simulink model "ctrl_custom"  (R2016b)
settings: Solver=ode3  StartTime=0.0  StopTime=inf  FixedStep=0.01  RelTol=1e-3  EnableMultiTasking=on
undefined symbols (not defined in the file): C, D, DiscIntNeverNeededParam, eps_c, epsilon, hd, hd2, I_s, k_cc, K_omega, K_q1f, K_q1r, K_q2f, K_q2r, K_q3f, K_q3r, K_q4f, K_q4r, K_q5f, K_q5r, K_q6f, K_q6r, K_T1f, K_T1r, K_T2f, K_T2r, K_T3f, K_T3r, K_T4f, K_T4r, K_T5f, K_T5r, K_T6f, K_T6r, Kp, Max_Acceleration, Max_rotation, Max_thrust, Min_thrust, n_c, n_max, p_cc, pwm_thr1_backward, pwm_thr1_forward, pwm_thr2_backward, pwm_thr2_forward, pwm_thr3_backward, pwm_thr3_forward, pwm_thr4_backward, pwm_thr4_forward, pwm_thr5_backward, pwm_thr5_forward, pwm_thr6_backward, pwm_thr6_forward, Q_f0, Q_max, r_cc, Rho, Thruster
libraries: dspmtrx3 x10, marine_gnc x8, simulink x7, simulink_extras x3
(part 4 of 6)

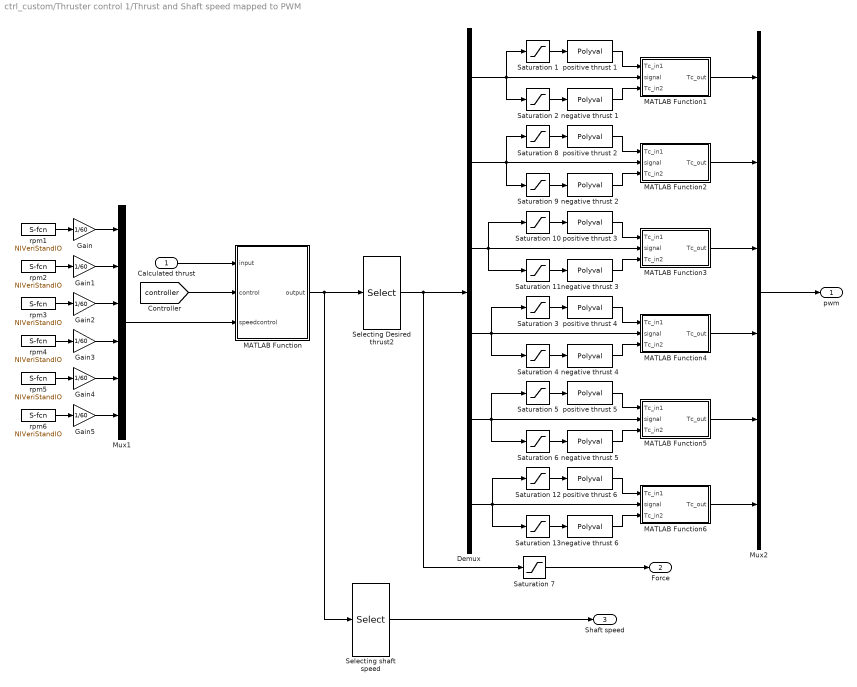
== system ctrl_custom/Thruster control 1/Thrust and Shaft speed mapped to PWM ==
  Calculated thrust : Inport
  Demux : Demux  Outputs=6
  Gain{,1..5} (6 alike) : Gain  Gain=1/60
  MATLAB Function : MATLAB Function  TreatAsAtomicUnit=on
  MATLAB Function1 : MATLAB Function  TreatAsAtomicUnit=on
  MATLAB Function2 : MATLAB Function  TreatAsAtomicUnit=on
  MATLAB Function3 : MATLAB Function  TreatAsAtomicUnit=on
  MATLAB Function4 : MATLAB Function  TreatAsAtomicUnit=on
  MATLAB Function5 : MATLAB Function  TreatAsAtomicUnit=on
  MATLAB Function6 : MATLAB Function  TreatAsAtomicUnit=on
  Mux1 : Mux  Inputs=6
  Mux2 : Mux  Inputs=6
  Saturation {1,3,5,8,10,12} (6 alike) : Saturate  UpperLimit=Max_thrust  LowerLimit=0
  Saturation {2,4,6,9,11,13} (6 alike) : Saturate  UpperLimit=0  LowerLimit=Min_thrust
  Saturation 7 : Saturate  UpperLimit=Max_thrust  LowerLimit=-Max_thrust
  Selecting Desired thrust2 : Selector  InputPortWidth=12  IndexOptions=Index vector (dialog)  Indices=[1 3 5 7 9 11]  OutputSizes=1
  Selecting shaft speed : Selector  InputPortWidth=12  IndexOptions=Index vector (dialog)  Indices=[2 4 6 8 10 12]  OutputSizes=1
  negative thrust 1 : Polyval  Coefs=pwm_thr1_backward
  negative thrust 2 : Polyval  Coefs=pwm_thr2_backward
  negative thrust 3 : Polyval  Coefs=pwm_thr3_backward
  negative thrust 4 : Polyval  Coefs=pwm_thr4_backward
  negative thrust 5 : Polyval  Coefs=pwm_thr5_backward
  negative thrust 6 : Polyval  Coefs=pwm_thr6_backward
  positive thrust 1 : Polyval  Coefs=pwm_thr1_forward
  positive thrust 2 : Polyval  Coefs=pwm_thr2_forward
  positive thrust 3 : Polyval  Coefs=pwm_thr3_forward
  positive thrust 4 : Polyval  Coefs=pwm_thr4_forward
  positive thrust 5 : Polyval  Coefs=pwm_thr5_forward
  positive thrust 6 : Polyval  Coefs=pwm_thr6_forward
  "rpm1 " : S-Function  Priority=1  FunctionName=NIVeriStandIO  Parameters=width dtype portnum stime stype btype  SFunctionDeploymentMode=off  EnableBusSupport=off  mask(NI VeriStand Inport){portnum=1, width=-1, stime=-1, dtype=auto, stype=auto, btype=1}
      mask prompts: portnum "Port number:"; width "Port dimensions (-1 for dynamically sized):"; stime "Sample time (-1 for inherited):"; dtype "Data type:"; stype "Signal type:"; btype "Block type:"
      mask help: Use this inport on any level of nested subsystems to allow NI VeriStand software to map signals to it.
      mask init:
      | NIVeriStandIO_init;
      settings: CopyFcn=NIVeriStand_MDL_functions('', 'IO_copy');  DeleteFcn=NIVeriStand_MDL_functions('', 'IO_delete');  MoveFcn=set_param(gcb, 'Mask', 'on');
      mask Callback portnum: NIVeriStand_MDL_functions('', 'IO_setportnum');
      mask TypeOptions dtype: auto | double | single | int8 | uint8 | int16 | uint16 | int32 | uint32 | boolean
      mask Callback dtype: NIVeriStand_MDL_functions('', 'IO_booleansignal');
      mask TypeOptions stype: auto | real | complex
      mask Display:
      | patch([-x x], [-y y], [.90980 .81960 .32156]);
      | plot([xrad -x x xrad], [yrad -y y yrad]);
      | fprintf('NI In%d', portnum);
  rpm2 : S-Function  Priority=2  FunctionName=NIVeriStandIO  Parameters=width dtype portnum stime stype btype  SFunctionDeploymentMode=off  EnableBusSupport=off  mask(NI VeriStand Inport){portnum=2, width=-1, stime=-1, dtype=auto, stype=auto, btype=1}
      mask prompts: portnum "Port number:"; width "Port dimensions (-1 for dynamically sized):"; stime "Sample time (-1 for inherited):"; dtype "Data type:"; stype "Signal type:"; btype "Block type:"
      mask help: Use this inport on any level of nested subsystems to allow NI VeriStand software to map signals to it.
      mask init:
      | NIVeriStandIO_init;
      settings: CopyFcn=NIVeriStand_MDL_functions('', 'IO_copy');  DeleteFcn=NIVeriStand_MDL_functions('', 'IO_delete');  MoveFcn=set_param(gcb, 'Mask', 'on');
      mask Callback portnum: NIVeriStand_MDL_functions('', 'IO_setportnum');
      mask TypeOptions dtype: auto | double | single | int8 | uint8 | int16 | uint16 | int32 | uint32 | boolean
      mask Callback dtype: NIVeriStand_MDL_functions('', 'IO_booleansignal');
      mask TypeOptions stype: auto | real | complex
      mask Display:
      | patch([-x x], [-y y], [.90980 .81960 .32156]);
      | plot([xrad -x x xrad], [yrad -y y yrad]);
      | fprintf('NI In%d', portnum);
  rpm3 : S-Function  Priority=3  FunctionName=NIVeriStandIO  Parameters=width dtype portnum stime stype btype  SFunctionDeploymentMode=off  EnableBusSupport=off  mask(NI VeriStand Inport){portnum=3, width=-1, stime=-1, dtype=auto, stype=auto, btype=1}
      mask prompts: portnum "Port number:"; width "Port dimensions (-1 for dynamically sized):"; stime "Sample time (-1 for inherited):"; dtype "Data type:"; stype "Signal type:"; btype "Block type:"
      mask help: Use this inport on any level of nested subsystems to allow NI VeriStand software to map signals to it.
      mask init:
      | NIVeriStandIO_init;
      settings: CopyFcn=NIVeriStand_MDL_functions('', 'IO_copy');  DeleteFcn=NIVeriStand_MDL_functions('', 'IO_delete');  MoveFcn=set_param(gcb, 'Mask', 'on');
      mask Callback portnum: NIVeriStand_MDL_functions('', 'IO_setportnum');
      mask TypeOptions dtype: auto | double | single | int8 | uint8 | int16 | uint16 | int32 | uint32 | boolean
      mask Callback dtype: NIVeriStand_MDL_functions('', 'IO_booleansignal');
      mask TypeOptions stype: auto | real | complex
      mask Display:
      | patch([-x x], [-y y], [.90980 .81960 .32156]);
      | plot([xrad -x x xrad], [yrad -y y yrad]);
      | fprintf('NI In%d', portnum);
  rpm4 : S-Function  Priority=4  FunctionName=NIVeriStandIO  Parameters=width dtype portnum stime stype btype  SFunctionDeploymentMode=off  EnableBusSupport=off  mask(NI VeriStand Inport){portnum=4, width=-1, stime=-1, dtype=auto, stype=auto, btype=1}
      mask prompts: portnum "Port number:"; width "Port dimensions (-1 for dynamically sized):"; stime "Sample time (-1 for inherited):"; dtype "Data type:"; stype "Signal type:"; btype "Block type:"
      mask help: Use this inport on any level of nested subsystems to allow NI VeriStand software to map signals to it.
      mask init:
      | NIVeriStandIO_init;
      settings: CopyFcn=NIVeriStand_MDL_functions('', 'IO_copy');  DeleteFcn=NIVeriStand_MDL_functions('', 'IO_delete');  MoveFcn=set_param(gcb, 'Mask', 'on');
      mask Callback portnum: NIVeriStand_MDL_functions('', 'IO_setportnum');
      mask TypeOptions dtype: auto | double | single | int8 | uint8 | int16 | uint16 | int32 | uint32 | boolean
      mask Callback dtype: NIVeriStand_MDL_functions('', 'IO_booleansignal');
      mask TypeOptions stype: auto | real | complex
      mask Display:
      | patch([-x x], [-y y], [.90980 .81960 .32156]);
      | plot([xrad -x x xrad], [yrad -y y yrad]);
      | fprintf('NI In%d', portnum);
  rpm5 : S-Function  Priority=5  FunctionName=NIVeriStandIO  Parameters=width dtype portnum stime stype btype  SFunctionDeploymentMode=off  EnableBusSupport=off  mask(NI VeriStand Inport){portnum=5, width=-1, stime=-1, dtype=auto, stype=auto, btype=1}
      mask prompts: portnum "Port number:"; width "Port dimensions (-1 for dynamically sized):"; stime "Sample time (-1 for inherited):"; dtype "Data type:"; stype "Signal type:"; btype "Block type:"
      mask help: Use this inport on any level of nested subsystems to allow NI VeriStand software to map signals to it.
      mask init:
      | NIVeriStandIO_init;
      settings: CopyFcn=NIVeriStand_MDL_functions('', 'IO_copy');  DeleteFcn=NIVeriStand_MDL_functions('', 'IO_delete');  MoveFcn=set_param(gcb, 'Mask', 'on');
      mask Callback portnum: NIVeriStand_MDL_functions('', 'IO_setportnum');
      mask TypeOptions dtype: auto | double | single | int8 | uint8 | int16 | uint16 | int32 | uint32 | boolean
      mask Callback dtype: NIVeriStand_MDL_functions('', 'IO_booleansignal');
      mask TypeOptions stype: auto | real | complex
      mask Display:
      | patch([-x x], [-y y], [.90980 .81960 .32156]);
      | plot([xrad -x x xrad], [yrad -y y yrad]);
      | fprintf('NI In%d', portnum);
  rpm6 : S-Function  Priority=6  FunctionName=NIVeriStandIO  Parameters=width dtype portnum stime stype btype  SFunctionDeploymentMode=off  EnableBusSupport=off  mask(NI VeriStand Inport){portnum=6, width=-1, stime=-1, dtype=auto, stype=auto, btype=1}
      mask prompts: portnum "Port number:"; width "Port dimensions (-1 for dynamically sized):"; stime "Sample time (-1 for inherited):"; dtype "Data type:"; stype "Signal type:"; btype "Block type:"
      mask help: Use this inport on any level of nested subsystems to allow NI VeriStand software to map signals to it.
      mask init:
      | NIVeriStandIO_init;
      settings: CopyFcn=NIVeriStand_MDL_functions('', 'IO_copy');  DeleteFcn=NIVeriStand_MDL_functions('', 'IO_delete');  MoveFcn=set_param(gcb, 'Mask', 'on');
      mask Callback portnum: NIVeriStand_MDL_functions('', 'IO_setportnum');
      mask TypeOptions dtype: auto | double | single | int8 | uint8 | int16 | uint16 | int32 | uint32 | boolean
      mask Callback dtype: NIVeriStand_MDL_functions('', 'IO_booleansignal');
      mask TypeOptions stype: auto | real | complex
      mask Display:
      | patch([-x x], [-y y], [.90980 .81960 .32156]);
      | plot([xrad -x x xrad], [yrad -y y yrad]);
      | fprintf('NI In%d', portnum);
  pwm : Outport
  Force : Outport  Port=2
  "Shaft speed " : Outport  Port=3
  wires:
  MATLAB Function/1(output) -> Selecting shaft speed/1, Selecting Desired thrust2/1
  [controller] -> MATLAB Function/2(control)
  Mux2/1 -> pwm/1
  Selecting Desired thrust2/1 -> Saturation 7/1, Demux/1
  Selecting shaft speed/1 -> "Shaft speed "/1
  Saturation 7/1 -> Force/1
  "rpm1 "/1 -> Gain/1
  rpm2/1 -> Gain1/1
  rpm3/1 -> Gain2/1
  rpm4/1 -> Gain3/1
  rpm5/1 -> Gain4/1
  rpm6/1 -> Gain5/1
  Mux1/1 -> MATLAB Function/3(speedcontrol)
  positive thrust 1/1 -> MATLAB Function1/1(Tc_in1)
  negative thrust 1/1 -> MATLAB Function1/3(Tc_in2)
  Demux/1 -> Saturation 1/1, MATLAB Function1/2(signal), Saturation 2/1
  MATLAB Function1/1(Tc_out) -> Mux2/1
  Saturation 1/1 -> positive thrust 1/1
  Saturation 2/1 -> negative thrust 1/1
  positive thrust 2/1 -> MATLAB Function2/1(Tc_in1)
  negative thrust 2/1 -> MATLAB Function2/3(Tc_in2)
  Demux/2 -> Saturation 9/1, Saturation 8/1, MATLAB Function2/2(signal)
  MATLAB Function2/1(Tc_out) -> Mux2/2
  Saturation 8/1 -> positive thrust 2/1
  Saturation 9/1 -> negative thrust 2/1
  positive thrust 3/1 -> MATLAB Function3/1(Tc_in1)
  negative thrust 3/1 -> MATLAB Function3/3(Tc_in2)
  Demux/3 -> Saturation 11/1, MATLAB Function3/2(signal), Saturation 10/1
  MATLAB Function3/1(Tc_out) -> Mux2/3
  Saturation 10/1 -> positive thrust 3/1
  Saturation 11/1 -> negative thrust 3/1
  positive thrust 4/1 -> MATLAB Function4/1(Tc_in1)
  negative thrust 4/1 -> MATLAB Function4/3(Tc_in2)
  MATLAB Function4/1(Tc_out) -> Mux2/4
  Saturation 3/1 -> positive thrust 4/1
  Saturation 4/1 -> negative thrust 4/1
  Demux/4 -> Saturation 3/1, Saturation 4/1, MATLAB Function4/2(signal)
  positive thrust 5/1 -> MATLAB Function5/1(Tc_in1)
  negative thrust 5/1 -> MATLAB Function5/3(Tc_in2)
  MATLAB Function5/1(Tc_out) -> Mux2/5
  Saturation 5/1 -> positive thrust 5/1
  Saturation 6/1 -> negative thrust 5/1
  Demux/5 -> Saturation 5/1, MATLAB Function5/2(signal), Saturation 6/1
  positive thrust 6/1 -> MATLAB Function6/1(Tc_in1)
  negative thrust 6/1 -> MATLAB Function6/3(Tc_in2)
  MATLAB Function6/1(Tc_out) -> Mux2/6
  Saturation 12/1 -> positive thrust 6/1
  Saturation 13/1 -> negative thrust 6/1
  Demux/6 -> Saturation 13/1, Saturation 12/1, MATLAB Function6/2(signal)
  Gain/1 -> Mux1/1
  Gain5/1 -> Mux1/6
  Gain4/1 -> Mux1/5
  Gain3/1 -> Mux1/4
  Gain2/1 -> Mux1/3
  Gain1/1 -> Mux1/2
  Calculated thrust/1 -> MATLAB Function/1(input)

== system ctrl_custom/Thruster control 1/Thruster 1 ==
  Desired thrust 1 : Inport
  shaft speed : Inport  Port=2
  Constant : Constant  Value=hd2.den{1,1}
  Constant1 : Constant  Value=hd2.num{1,1}
  Delay : Delay  DelayLength=1  InitialCondition=0
  Discrete Transfer Fcn : DiscreteTransferFcn  NumeratorSource=Input port  DenominatorSource=Input port  Denominator=[0.2 1]  SampleTime=0.01  a0EqualsOne=on
      settings: InputPortMap=u0,p1,p3
  Losses (placeholder) : Constant  Value=0
  Propeller Hydrodynamics : Subsystem
  Shaft dynamics : Subsystem
  Thruster control : Subsystem
  "Commanded thrust " : Outport
  Shaft speed : Outport  Port=2
  wires:
  Losses (placeholder)/1 -> Propeller Hydrodynamics/1(env)
  Shaft dynamics/1(n) -> Shaft speed/1, Propeller Hydrodynamics/2(n)
  Propeller Hydrodynamics/2(Qa) -> Delay/1
  Propeller Hydrodynamics/1(Ta) -> "Commanded thrust "/1
  Thruster control/1(Qc) -> Discrete Transfer Fcn/1
  Constant1/1 -> Discrete Transfer Fcn/2
  Constant/1 -> Discrete Transfer Fcn/3
  Discrete Transfer Fcn/1 -> Shaft dynamics/1(Qm)
  shaft speed/1 -> Thruster control/2(n)
  Delay/1 -> Shaft dynamics/2(Qa)
  Desired thrust 1/1 -> Thruster control/1("T_d ")

== system ctrl_custom/Thruster control 1/Thruster 2 ==
  Desired thrust 1 : Inport
  shaft speed : Inport  Port=2
  Constant : Constant  Value=hd2.den{1,1}
  Constant1 : Constant  Value=hd2.num{1,1}
  Delay : Delay  DelayLength=1  InitialCondition=0
  Discrete Transfer Fcn : DiscreteTransferFcn  NumeratorSource=Input port  DenominatorSource=Input port  Denominator=[0.2 1]  SampleTime=0.01  a0EqualsOne=on
      settings: InputPortMap=u0,p1,p3
  Losses (placeholder) : Constant  Value=0
  Propeller Hydrodynamics : Subsystem
  Shaft dynamics : Subsystem
  Thruster control : Subsystem
  "Commanded thrust " : Outport
  Shaft speed : Outport  Port=2
  wires:
  Losses (placeholder)/1 -> Propeller Hydrodynamics/1(env)
  Shaft dynamics/1(n) -> Propeller Hydrodynamics/2(n), Shaft speed/1
  Propeller Hydrodynamics/2(Qa) -> Delay/1
  Thruster control/1(Qc) -> Discrete Transfer Fcn/1
  Discrete Transfer Fcn/1 -> Shaft dynamics/1(Qm)
  Desired thrust 1/1 -> Thruster control/1("T_d ")
  Propeller Hydrodynamics/1(Ta) -> "Commanded thrust "/1
  Constant1/1 -> Discrete Transfer Fcn/2
  Constant/1 -> Discrete Transfer Fcn/3
  shaft speed/1 -> Thruster control/2(n)
  Delay/1 -> Shaft dynamics/2(Qa)

== system ctrl_custom/Thruster control 1/Thruster 3 ==
  Desired thrust 1 : Inport
  shaft speed : Inport  Port=2
  Constant : Constant  Value=hd2.den{1,1}
  Constant1 : Constant  Value=hd2.num{1,1}
  Delay : Delay  DelayLength=1  InitialCondition=0
  Discrete Transfer Fcn : DiscreteTransferFcn  NumeratorSource=Input port  DenominatorSource=Input port  Denominator=[0.2 1]  SampleTime=0.01  a0EqualsOne=on
      settings: InputPortMap=u0,p1,p3
  Losses (placeholder) : Constant  Value=0
  Propeller Hydrodynamics : Subsystem
  Shaft dynamics : Subsystem
  Thruster control : Subsystem
  "Commanded thrust " : Outport
  Shaft speed : Outport  Port=2
  wires:
  Losses (placeholder)/1 -> Propeller Hydrodynamics/1(env)
  Shaft dynamics/1(n) -> Propeller Hydrodynamics/2(n), Shaft speed/1
  Propeller Hydrodynamics/2(Qa) -> Delay/1
  Thruster control/1(Qc) -> Discrete Transfer Fcn/1
  Discrete Transfer Fcn/1 -> Shaft dynamics/1(Qm)
  Desired thrust 1/1 -> Thruster control/1("T_d ")
  Propeller Hydrodynamics/1(Ta) -> "Commanded thrust "/1
  Constant1/1 -> Discrete Transfer Fcn/2
  Constant/1 -> Discrete Transfer Fcn/3
  shaft speed/1 -> Thruster control/2(n)
  Delay/1 -> Shaft dynamics/2(Qa)

== system ctrl_custom/Thruster control 1/Thruster 4 ==
  Desired thrust 1 : Inport
  shaft speed : Inport  Port=2
  Constant : Constant  Value=hd2.den{1,1}
  Constant1 : Constant  Value=hd2.num{1,1}
  Delay : Delay  DelayLength=1  InitialCondition=0
  Discrete Transfer Fcn : DiscreteTransferFcn  NumeratorSource=Input port  DenominatorSource=Input port  Denominator=[0.2 1]  SampleTime=0.01  a0EqualsOne=on
      settings: InputPortMap=u0,p1,p3
  Losses (placeholder) : Constant  Value=0
  Propeller Hydrodynamics : Subsystem
  Shaft dynamics : Subsystem
  Thruster control : Subsystem
  "Commanded thrust " : Outport
  Shaft speed : Outport  Port=2
  wires:
  Losses (placeholder)/1 -> Propeller Hydrodynamics/1(env)
  Shaft dynamics/1(n) -> Propeller Hydrodynamics/2(n), Shaft speed/1
  Propeller Hydrodynamics/2(Qa) -> Delay/1
  Thruster control/1(Qc) -> Discrete Transfer Fcn/1
  Discrete Transfer Fcn/1 -> Shaft dynamics/1(Qm)
  Desired thrust 1/1 -> Thruster control/1("T_d ")
  Propeller Hydrodynamics/1(Ta) -> "Commanded thrust "/1
  Constant1/1 -> Discrete Transfer Fcn/2
  Constant/1 -> Discrete Transfer Fcn/3
  shaft speed/1 -> Thruster control/2(n)
  Delay/1 -> Shaft dynamics/2(Qa)

== system ctrl_custom/Thruster control 1/Thruster 5 ==
  Desired thrust 1 : Inport
  shaft speed : Inport  Port=2
  Constant : Constant  Value=hd2.den{1,1}
  Constant1 : Constant  Value=hd2.num{1,1}
  Delay : Delay  DelayLength=1  InitialCondition=0
  Discrete Transfer Fcn : DiscreteTransferFcn  NumeratorSource=Input port  DenominatorSource=Input port  Denominator=[0.2 1]  SampleTime=0.01  a0EqualsOne=on
      settings: InputPortMap=u0,p1,p3
  Losses (placeholder) : Constant  Value=0
  Propeller Hydrodynamics : Subsystem
  Shaft dynamics : Subsystem
  Thruster control : Subsystem
  "Commanded thrust " : Outport
  Shaft speed : Outport  Port=2
  wires:
  Losses (placeholder)/1 -> Propeller Hydrodynamics/1(env)
  Shaft dynamics/1(n) -> Propeller Hydrodynamics/2(n), Shaft speed/1
  Propeller Hydrodynamics/2(Qa) -> Delay/1
  Thruster control/1(Qc) -> Discrete Transfer Fcn/1
  Discrete Transfer Fcn/1 -> Shaft dynamics/1(Qm)
  Desired thrust 1/1 -> Thruster control/1("T_d ")
  Propeller Hydrodynamics/1(Ta) -> "Commanded thrust "/1
  Constant1/1 -> Discrete Transfer Fcn/2
  Constant/1 -> Discrete Transfer Fcn/3
  shaft speed/1 -> Thruster control/2(n)
  Delay/1 -> Shaft dynamics/2(Qa)

== system ctrl_custom/Thruster control 1/Thruster 6 ==
  Desired thrust 1 : Inport
  shaft speed : Inport  Port=2
  Constant : Constant  Value=hd2.den{1,1}
  Constant1 : Constant  Value=hd2.num{1,1}
  Delay : Delay  DelayLength=1  InitialCondition=0
  Discrete Transfer Fcn : DiscreteTransferFcn  NumeratorSource=Input port  DenominatorSource=Input port  Denominator=[0.2 1]  SampleTime=0.01  a0EqualsOne=on
      settings: InputPortMap=u0,p1,p3
  Losses (placeholder) : Constant  Value=0
  Propeller Hydrodynamics : Subsystem
  Shaft dynamics : Subsystem
  Thruster control : Subsystem
  "Commanded thrust " : Outport
  Shaft speed : Outport  Port=2
  wires:
  Losses (placeholder)/1 -> Propeller Hydrodynamics/1(env)
  Shaft dynamics/1(n) -> Propeller Hydrodynamics/2(n), Shaft speed/1
  Propeller Hydrodynamics/2(Qa) -> Delay/1
  Thruster control/1(Qc) -> Discrete Transfer Fcn/1
  Discrete Transfer Fcn/1 -> Shaft dynamics/1(Qm)
  Desired thrust 1/1 -> Thruster control/1("T_d ")
  Propeller Hydrodynamics/1(Ta) -> "Commanded thrust "/1
  Constant1/1 -> Discrete Transfer Fcn/2
  Constant/1 -> Discrete Transfer Fcn/3
  shaft speed/1 -> Thruster control/2(n)
  Delay/1 -> Shaft dynamics/2(Qa)

== system ctrl_custom/Thruster control 1/Thruster 1/Propeller Hydrodynamics ==
  env : Inport
  n : Inport  Port=2
  Actual Force and Torque : MATLAB Function  TreatAsAtomicUnit=on
  Control_test_Pa : S-Function  Priority=1  FunctionName=NIVeriStandIO  Parameters=width dtype portnum stime stype btype  SFunctionDeploymentMode=off  EnableBusSupport=off  mask(NI VeriStand Outport){portnum=1, width=-1, stime=-1, dtype=auto, stype=auto, btype=0}
      mask prompts: portnum "Port number:"; width "Port dimensions (-1 for dynamically sized):"; stime "Sample time (-1 for inherited):"; dtype "Data type:"; stype "Signal type:"; btype "Block type:"
      mask help: Use this outport on any level of nested subsystems to allow NI VeriStand software to map signals to it.
      mask init:
      | NIVeriStandIO_init;
      settings: CopyFcn=NIVeriStand_MDL_functions('', 'IO_copy');  DeleteFcn=NIVeriStand_MDL_functions('', 'IO_delete');  MoveFcn=set_param(gcb, 'Mask', 'on');
      mask Callback portnum: NIVeriStand_MDL_functions('', 'IO_setportnum');
      mask TypeOptions dtype: auto | double | single | int8 | uint8 | int16 | uint16 | int32 | uint32 | boolean
      mask Callback dtype: NIVeriStand_MDL_functions('', 'IO_booleansignal');
      mask TypeOptions stype: auto | real | complex
      mask Display:
      | patch([-x x], [-y y], [.90980 .81960 .32156]);
      | plot([xrad -x x xrad], [yrad -y y yrad]);
      | fprintf('NI Out%d', portnum);
  Ta : Outport
  Qa : Outport  Port=2
  wires:
  n/1 -> Actual Force and Torque/1(n)
  [D] -> Actual Force and Torque/7(D)
  [Kq1f] -> Actual Force and Torque/2(Kq)
  Actual Force and Torque/2(Qa) -> Qa/1
  [Rho] -> Actual Force and Torque/6(Rho)
  env/1 -> Actual Force and Torque/9(env)
  [Kt1f] -> Actual Force and Torque/3(Kt)
  Actual Force and Torque/1(Ta) -> Ta/1
  [Kt1r] -> Actual Force and Torque/4(Ktr)
  [Kq1r] -> Actual Force and Torque/5(Kqr)
  [eps_c] -> Actual Force and Torque/8(eps_c)
  Actual Force and Torque/3(Pa) -> Control_test_Pa/1

== system ctrl_custom/Thruster control 1/Thruster 1/Shaft dynamics ==
  Qm : Inport
  Qa : Inport  Port=2
  Finding rotation speed : Gain  Gain=1/(2*pi*I_s)
  Integrator : Integrator  ExternalReset=either
  K_omega : Gain  Gain=K_omega*2*pi
  Sum : Sum  Inputs=-+-
  n : Outport
  wires:
  Qm/1 -> Sum/2
  Sum/1 -> Finding rotation speed/1
  Qa/1 -> Sum/1
  K_omega/1 -> Sum/3
  Finding rotation speed/1 -> Integrator/1
  Integrator/1 -> K_omega/1, n/1
  [reset] -> Integrator/2

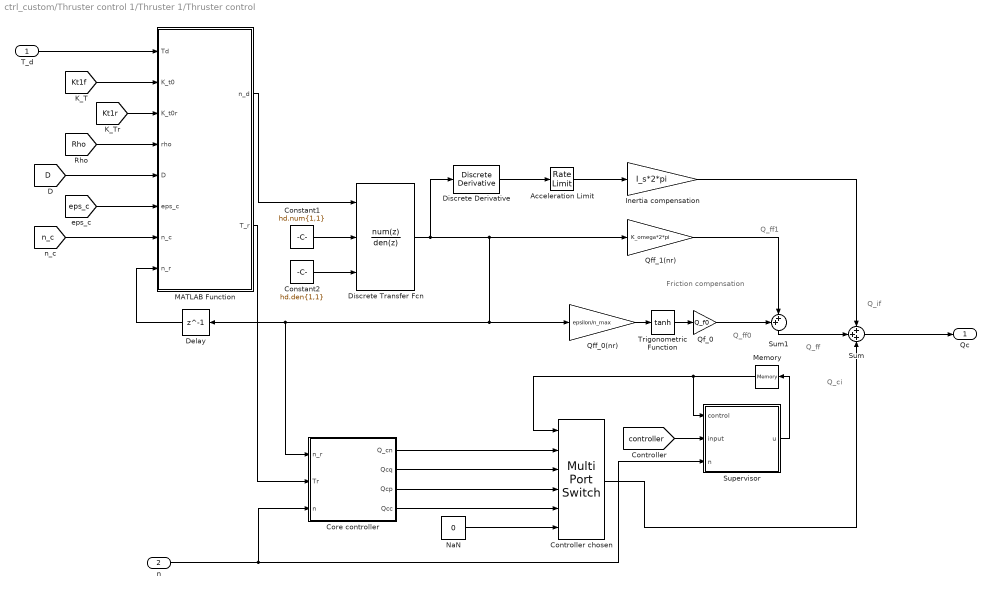
== system ctrl_custom/Thruster control 1/Thruster 1/Thruster control ==
  note: Q_ci
  note: Q_if
  note: Q_ff
  note: Q_ff0
  note: Q_ff1
  note: Friction compensation
  "T_d " : Inport
  n : Inport  Port=2
  Acceleration Limit : RateLimiter  RisingSlewLimit=Max_Acceleration  FallingSlewLimit=-Max_Acceleration  SampleTimeMode=inherited
  Constant1 : Constant  Value=hd.num{1,1}  VectorParams1D=off
  Constant2 : Constant  Value=hd.den{1,1}  VectorParams1D=off
  Controller chosen : MultiPortSwitch  Inputs=5
  Core controller : Subsystem
  Delay : Delay  DelayLength=1  InitialCondition=0
  Discrete Transfer Fcn : DiscreteTransferFcn  NumeratorSource=Input port  Numerator=[8.76e-05 0.0003481 8.648e-05]  DenominatorSource=Input port  Denominator=[1 -1.974 0.9746]  SampleTime=0.01  a0EqualsOne=on
      settings: InputPortMap=u0,p1,p3
  Discrete Derivative : simulink/Discrete/Discrete Derivative  gainval=1.0  ICPrevScaledInput=0.0  InputProcessing=Inherited  OutMin=[]  OutMax=[]  OutDataType=fixdt(1, 16)  OutScaling=2^-10  DoSatur=off
  Inertia compensation : Gain  Gain=I_s*2*pi
  MATLAB Function : MATLAB Function  TreatAsAtomicUnit=on
  Memory : Memory  X0=1  InheritSampleTime=on
  NaN : Constant  Value=0
  Qf_0 : Gain  Gain=Q_f0
  Qff_0(nr) : Gain  Gain=epsilon/n_max
  Qff_1(nr) : Gain  Gain=K_omega*2*pi
  Sum : Sum  Inputs=+++
  Sum1 : Sum  Inputs=++|
  Supervisor : MATLAB Function  TreatAsAtomicUnit=on
  Trigonometric Function : Trigonometry  Operator=tanh
  Qc : Outport
  wires:
  "T_d "/1 -> MATLAB Function/1(Td)
  [Rho] -> MATLAB Function/4(rho)
  [D] -> MATLAB Function/5(D)
  [eps_c] -> MATLAB Function/6(eps_c)
  MATLAB Function/2(T_r) -> Core controller/2("Tr ")
  MATLAB Function/1(n_d) -> Discrete Transfer Fcn/1
  Qff_0(nr)/1 -> Trigonometric Function/1
  Trigonometric Function/1 -> Qf_0/1
  NaN/1 -> Controller chosen/6
  Supervisor/1(u) -> Memory/1
  Memory/1 -> Controller chosen/1, Supervisor/1(control)
  Qff_1(nr)/1 -> Sum1/2
  Qf_0/1 -> Sum1/1
  [controller] -> Supervisor/2(input)
  Controller chosen/1 -> Sum/3
  Sum/1 -> Qc/1
  Core controller/2(Qcq) -> Controller chosen/3
  Core controller/3(Qcp) -> Controller chosen/4
  Core controller/4(Qcc) -> Controller chosen/5
  Core controller/1(Q_cn) -> Controller chosen/2
  [n_c] -> MATLAB Function/7(n_c)
  Discrete Derivative/1 -> Acceleration Limit/1
  Sum1/1 -> Sum/2
  Constant1/1 -> Discrete Transfer Fcn/2
  Constant2/1 -> Discrete Transfer Fcn/3
  Inertia compensation/1 -> Sum/1
  n/1 -> Core controller/3("n "), Supervisor/3(n)
  Acceleration Limit/1 -> Inertia compensation/1
  Discrete Transfer Fcn/1 -> Core controller/1(n_r), Delay/1, Qff_0(nr)/1, Qff_1(nr)/1, Discrete Derivative/1
  Delay/1 -> MATLAB Function/8(n_r)
  [Kt1r] -> MATLAB Function/3(K_t0r)
  [Kt1f] -> MATLAB Function/2(K_t0)

== system ctrl_custom/Thruster control 1/Thruster 2/Propeller Hydrodynamics ==
  env : Inport
  n : Inport  Port=2
  Actual Force and Torque : MATLAB Function  TreatAsAtomicUnit=on
  Ta : Outport
  Qa : Outport  Port=2
  wires:
  n/1 -> Actual Force and Torque/1(n)
  [D] -> Actual Force and Torque/7(D)
  [Kq2f] -> Actual Force and Torque/2(Kq)
  Actual Force and Torque/2(Qa) -> Qa/1
  [Rho] -> Actual Force and Torque/6(Rho)
  env/1 -> Actual Force and Torque/9(env)
  [Kt2f] -> Actual Force and Torque/3(Kt)
  Actual Force and Torque/1(Ta) -> Ta/1
  [Kt2r] -> Actual Force and Torque/4(Ktr)
  [Kq2r] -> Actual Force and Torque/5(Kqr)
  [eps_c] -> Actual Force and Torque/8(eps_c)

== system ctrl_custom/Thruster control 1/Thruster 2/Shaft dynamics ==
  Qm : Inport
  Qa : Inport  Port=2
  Finding rotation speed : Gain  Gain=1/(2*pi*I_s)
  Integrator : Integrator  ExternalReset=either
  K_omega : Gain  Gain=K_omega*2*pi
  Sum : Sum  Inputs=-+-
  n : Outport
  wires:
  Qm/1 -> Sum/2
  Sum/1 -> Finding rotation speed/1
  Qa/1 -> Sum/1
  K_omega/1 -> Sum/3
  Finding rotation speed/1 -> Integrator/1
  Integrator/1 -> K_omega/1, n/1
  [reset] -> Integrator/2

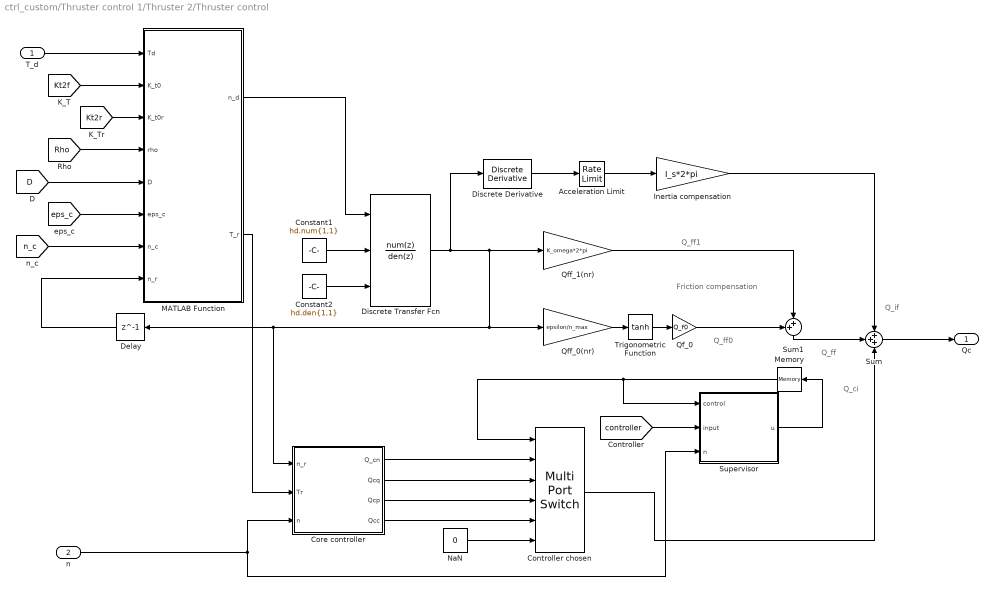
== system ctrl_custom/Thruster control 1/Thruster 2/Thruster control ==
  note: Q_ci
  note: Q_if
  note: Q_ff
  note: Q_ff0
  note: Q_ff1
  note: Friction compensation
  "T_d " : Inport
  n : Inport  Port=2
  Acceleration Limit : RateLimiter  RisingSlewLimit=Max_Acceleration  FallingSlewLimit=-Max_Acceleration  SampleTimeMode=inherited
  Constant1 : Constant  Value=hd.num{1,1}  VectorParams1D=off
  Constant2 : Constant  Value=hd.den{1,1}  VectorParams1D=off
  Controller chosen : MultiPortSwitch  Inputs=5
  Core controller : Subsystem
  Delay : Delay  DelayLength=1  InitialCondition=0
  Discrete Transfer Fcn : DiscreteTransferFcn  NumeratorSource=Input port  Numerator=[8.76e-05 0.0003481 8.648e-05]  DenominatorSource=Input port  Denominator=[1 -1.974 0.9746]  SampleTime=0.01  a0EqualsOne=on
      settings: InputPortMap=u0,p1,p3
  Discrete Derivative : simulink/Discrete/Discrete Derivative  gainval=1.0  ICPrevScaledInput=0.0  InputProcessing=Inherited  OutMin=[]  OutMax=[]  OutDataType=fixdt(1, 16)  OutScaling=2^-10  DoSatur=off
  Inertia compensation : Gain  Gain=I_s*2*pi
  MATLAB Function : MATLAB Function  TreatAsAtomicUnit=on
  Memory : Memory  X0=1
  NaN : Constant  Value=0
  Qf_0 : Gain  Gain=Q_f0
  Qff_0(nr) : Gain  Gain=epsilon/n_max
  Qff_1(nr) : Gain  Gain=K_omega*2*pi
  Sum : Sum  Inputs=+++
  Sum1 : Sum  Inputs=++|
  Supervisor : MATLAB Function  TreatAsAtomicUnit=on
  Trigonometric Function : Trigonometry  Operator=tanh
  Qc : Outport
  wires:
  Sum/1 -> Qc/1
  MATLAB Function/2(T_r) -> Core controller/2("Tr ")
  Qff_0(nr)/1 -> Trigonometric Function/1
  Trigonometric Function/1 -> Qf_0/1
  Sum1/1 -> Sum/2
  Core controller/1(Q_cn) -> Controller chosen/2
  Core controller/4(Qcc) -> Controller chosen/5
  NaN/1 -> Controller chosen/6
  Memory/1 -> Supervisor/1(control), Controller chosen/1
  Qff_1(nr)/1 -> Sum1/2
  Qf_0/1 -> Sum1/1
  Controller chosen/1 -> Sum/3
  Inertia compensation/1 -> Sum/1
  Core controller/3(Qcp) -> Controller chosen/4
  Core controller/2(Qcq) -> Controller chosen/3
  [controller] -> Supervisor/2(input)
  "T_d "/1 -> MATLAB Function/1(Td)
  [Rho] -> MATLAB Function/4(rho)
  [D] -> MATLAB Function/5(D)
  [eps_c] -> MATLAB Function/6(eps_c)
  [n_c] -> MATLAB Function/7(n_c)
  Constant1/1 -> Discrete Transfer Fcn/2
  Constant2/1 -> Discrete Transfer Fcn/3
  MATLAB Function/1(n_d) -> Discrete Transfer Fcn/1
  Discrete Derivative/1 -> Acceleration Limit/1
  n/1 -> Supervisor/3(n), Core controller/3("n ")
  Discrete Transfer Fcn/1 -> Discrete Derivative/1, Qff_0(nr)/1, Core controller/1(n_r), Delay/1, Qff_1(nr)/1
  Acceleration Limit/1 -> Inertia compensation/1
  Supervisor/1(u) -> Memory/1
  Delay/1 -> MATLAB Function/8(n_r)
  [Kt2r] -> MATLAB Function/3(K_t0r)
  [Kt2f] -> MATLAB Function/2(K_t0)

== system ctrl_custom/Thruster control 1/Thruster 3/Propeller Hydrodynamics ==
  env : Inport
  n : Inport  Port=2
  Actual Force and Torque : MATLAB Function  TreatAsAtomicUnit=on
  Ta : Outport
  Qa : Outport  Port=2
  wires:
  n/1 -> Actual Force and Torque/1(n)
  [D] -> Actual Force and Torque/7(D)
  [Kq3f] -> Actual Force and Torque/2(Kq)
  Actual Force and Torque/2(Qa) -> Qa/1
  [Rho] -> Actual Force and Torque/6(Rho)
  env/1 -> Actual Force and Torque/9(env)
  [Kt3f] -> Actual Force and Torque/3(Kt)
  Actual Force and Torque/1(Ta) -> Ta/1
  [Kt3r] -> Actual Force and Torque/4(Ktr)
  [Kq3r] -> Actual Force and Torque/5(Kqr)
  [eps_c] -> Actual Force and Torque/8(eps_c)

== system ctrl_custom/Thruster control 1/Thruster 3/Shaft dynamics ==
  Qm : Inport
  Qa : Inport  Port=2
  Finding rotation speed : Gain  Gain=1/(2*pi*I_s)
  Integrator : Integrator  ExternalReset=either
  K_omega : Gain  Gain=K_omega*2*pi
  Sum : Sum  Inputs=-+-
  n : Outport
  wires:
  Qm/1 -> Sum/2
  Sum/1 -> Finding rotation speed/1
  Qa/1 -> Sum/1
  K_omega/1 -> Sum/3
  Finding rotation speed/1 -> Integrator/1
  Integrator/1 -> n/1, K_omega/1
  [reset] -> Integrator/2

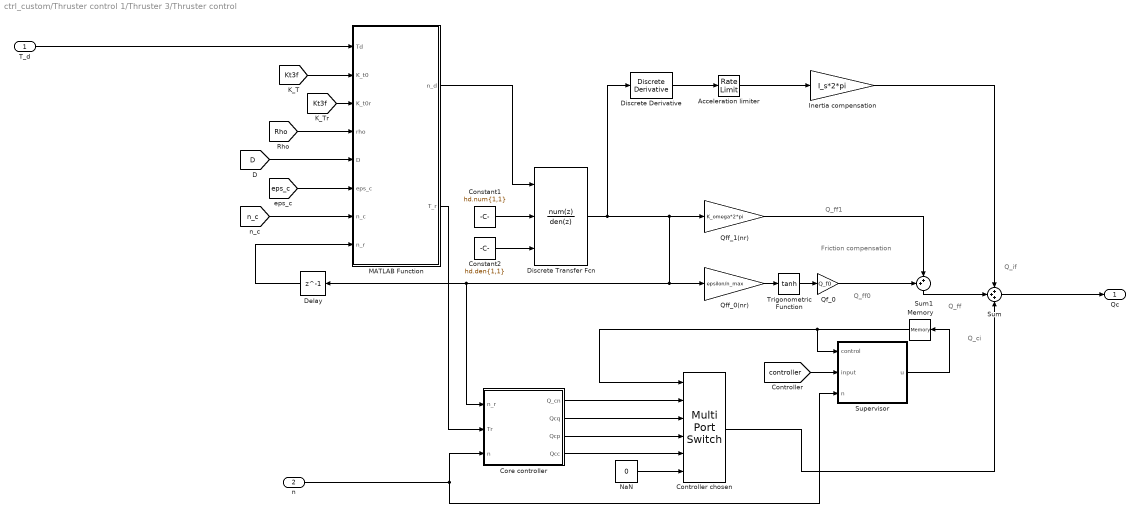
== system ctrl_custom/Thruster control 1/Thruster 3/Thruster control ==
  note: Q_ci
  note: Q_if
  note: Q_ff
  note: Q_ff0
  note: Q_ff1
  note: Friction compensation
  "T_d " : Inport
  n : Inport  Port=2
  Acceleration limiter : RateLimiter  RisingSlewLimit=Max_Acceleration  FallingSlewLimit=-Max_Acceleration  SampleTimeMode=inherited
  Constant1 : Constant  Value=hd.num{1,1}  VectorParams1D=off
  Constant2 : Constant  Value=hd.den{1,1}  VectorParams1D=off
  Controller chosen : MultiPortSwitch  Inputs=5
  Core controller : Subsystem
  Delay : Delay  DelayLength=1  InitialCondition=0
  Discrete Transfer Fcn : DiscreteTransferFcn  NumeratorSource=Input port  Numerator=[8.76e-05 0.0003481 8.648e-05]  DenominatorSource=Input port  Denominator=[1 -1.974 0.9746]  SampleTime=0.01  a0EqualsOne=on
      settings: InputPortMap=u0,p1,p3
  Discrete Derivative : simulink/Discrete/Discrete Derivative  gainval=1.0  ICPrevScaledInput=0.0  InputProcessing=Inherited  OutMin=[]  OutMax=[]  OutDataType=fixdt(1, 16)  OutScaling=2^-10  DoSatur=off
  Inertia compensation : Gain  Gain=I_s*2*pi
  MATLAB Function : MATLAB Function  TreatAsAtomicUnit=on
  Memory : Memory  X0=1
  NaN : Constant  Value=0
  Qf_0 : Gain  Gain=Q_f0
  Qff_0(nr) : Gain  Gain=epsilon/n_max
  Qff_1(nr) : Gain  Gain=K_omega*2*pi
  Sum : Sum  Inputs=+++
  Sum1 : Sum  Inputs=++|
  Supervisor : MATLAB Function  TreatAsAtomicUnit=on
  Trigonometric Function : Trigonometry  Operator=tanh
  Qc : Outport
  wires:
  Sum/1 -> Qc/1
  MATLAB Function/2(T_r) -> Core controller/2("Tr ")
  Discrete Derivative/1 -> Acceleration limiter/1
  Qff_0(nr)/1 -> Trigonometric Function/1
  Trigonometric Function/1 -> Qf_0/1
  Sum1/1 -> Sum/2
  Core controller/1(Q_cn) -> Controller chosen/2
  Core controller/4(Qcc) -> Controller chosen/5
  NaN/1 -> Controller chosen/6
  Memory/1 -> Controller chosen/1, Supervisor/1(control)
  Qff_1(nr)/1 -> Sum1/2
  Qf_0/1 -> Sum1/1
  Controller chosen/1 -> Sum/3
  Inertia compensation/1 -> Sum/1
  Core controller/3(Qcp) -> Controller chosen/4
  Core controller/2(Qcq) -> Controller chosen/3
  [controller] -> Supervisor/2(input)
  "T_d "/1 -> MATLAB Function/1(Td)
  [Rho] -> MATLAB Function/4(rho)
  [D] -> MATLAB Function/5(D)
  [eps_c] -> MATLAB Function/6(eps_c)
  [n_c] -> MATLAB Function/7(n_c)
  Constant1/1 -> Discrete Transfer Fcn/2
  Constant2/1 -> Discrete Transfer Fcn/3
  MATLAB Function/1(n_d) -> Discrete Transfer Fcn/1
  n/1 -> Supervisor/3(n), Core controller/3("n ")
  Discrete Transfer Fcn/1 -> Discrete Derivative/1, Core controller/1(n_r), Delay/1, Qff_0(nr)/1, Qff_1(nr)/1
  Acceleration limiter/1 -> Inertia compensation/1
  Supervisor/1(u) -> Memory/1
  Delay/1 -> MATLAB Function/8(n_r)
  [Kt3f] -> MATLAB Function/3(K_t0r)
  [Kt3f] -> MATLAB Function/2(K_t0)

== system ctrl_custom/Thruster control 1/Thruster 4/Propeller Hydrodynamics ==
  env : Inport
  n : Inport  Port=2
  Actual Force and Torque : MATLAB Function  TreatAsAtomicUnit=on
  Ta : Outport
  Qa : Outport  Port=2
  wires:
  n/1 -> Actual Force and Torque/1(n)
  [D] -> Actual Force and Torque/7(D)
  [Kq4f] -> Actual Force and Torque/2(Kq)
  Actual Force and Torque/2(Qa) -> Qa/1
  [Rho] -> Actual Force and Torque/6(Rho)
  env/1 -> Actual Force and Torque/9(env)
  [Kt4f] -> Actual Force and Torque/3(Kt)
  Actual Force and Torque/1(Ta) -> Ta/1
  [Kt4r] -> Actual Force and Torque/4(Ktr)
  [Kq4r] -> Actual Force and Torque/5(Kqr)
  [eps_c] -> Actual Force and Torque/8(eps_c)

== system ctrl_custom/Thruster control 1/Thruster 4/Shaft dynamics ==
  Qm : Inport
  Qa : Inport  Port=2
  Finding rotation speed : Gain  Gain=1/(2*pi*I_s)
  Integrator : Integrator  ExternalReset=either
  K_omega : Gain  Gain=K_omega*2*pi
  Sum : Sum  Inputs=-+-
  n : Outport
  wires:
  Qm/1 -> Sum/2
  Sum/1 -> Finding rotation speed/1
  Qa/1 -> Sum/1
  K_omega/1 -> Sum/3
  Finding rotation speed/1 -> Integrator/1
  Integrator/1 -> K_omega/1, n/1
  [reset] -> Integrator/2

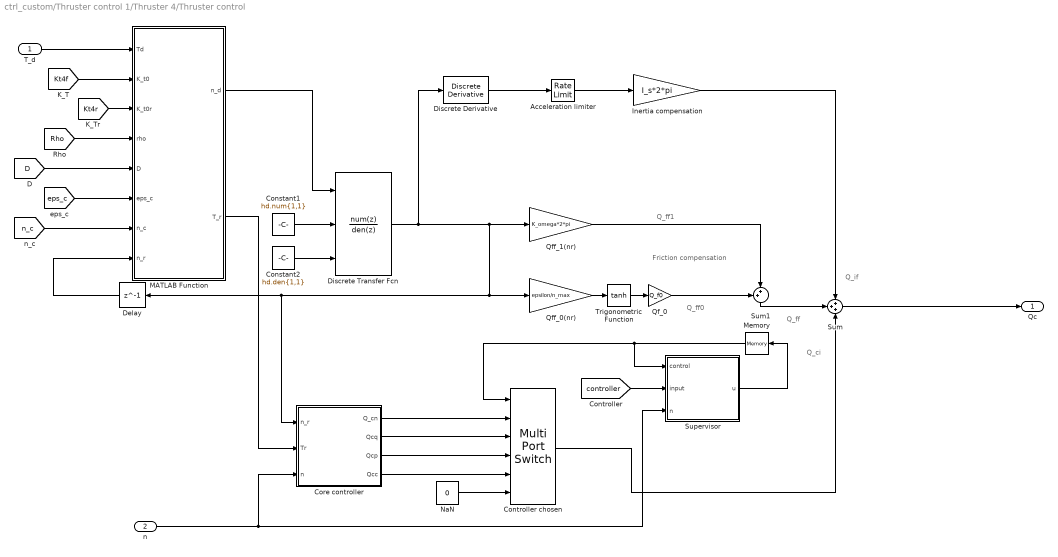
== system ctrl_custom/Thruster control 1/Thruster 4/Thruster control ==
  note: Q_ci
  note: Q_if
  note: Q_ff
  note: Q_ff0
  note: Q_ff1
  note: Friction compensation
  "T_d " : Inport
  n : Inport  Port=2
  Acceleration limiter : RateLimiter  RisingSlewLimit=Max_Acceleration  FallingSlewLimit=-Max_Acceleration  SampleTimeMode=inherited
  Constant1 : Constant  Value=hd.num{1,1}  VectorParams1D=off
  Constant2 : Constant  Value=hd.den{1,1}  VectorParams1D=off
  Controller chosen : MultiPortSwitch  Inputs=5
  Core controller : Subsystem
  Delay : Delay  DelayLength=1  InitialCondition=0
  Discrete Transfer Fcn : DiscreteTransferFcn  NumeratorSource=Input port  Numerator=[8.76e-05 0.0003481 8.648e-05]  DenominatorSource=Input port  Denominator=[1 -1.974 0.9746]  SampleTime=0.01  a0EqualsOne=on
      settings: InputPortMap=u0,p1,p3
  Discrete Derivative : simulink/Discrete/Discrete Derivative  gainval=1.0  ICPrevScaledInput=0.0  InputProcessing=Inherited  OutMin=[]  OutMax=[]  OutDataType=fixdt(1, 16)  OutScaling=2^-10  DoSatur=off
  Inertia compensation : Gain  Gain=I_s*2*pi
  MATLAB Function : MATLAB Function  TreatAsAtomicUnit=on
  Memory : Memory  X0=1
  NaN : Constant  Value=0
  Qf_0 : Gain  Gain=Q_f0
  Qff_0(nr) : Gain  Gain=epsilon/n_max
  Qff_1(nr) : Gain  Gain=K_omega*2*pi
  Sum : Sum  Inputs=+++
  Sum1 : Sum  Inputs=++|
  Supervisor : MATLAB Function  TreatAsAtomicUnit=on
  Trigonometric Function : Trigonometry  Operator=tanh
  Qc : Outport
  wires:
  Sum/1 -> Qc/1
  MATLAB Function/2(T_r) -> Core controller/2("Tr ")
  Discrete Derivative/1 -> Acceleration limiter/1
  Qff_0(nr)/1 -> Trigonometric Function/1
  Trigonometric Function/1 -> Qf_0/1
  Sum1/1 -> Sum/2
  Core controller/1(Q_cn) -> Controller chosen/2
  Core controller/4(Qcc) -> Controller chosen/5
  NaN/1 -> Controller chosen/6
  Memory/1 -> Controller chosen/1, Supervisor/1(control)
  Qff_1(nr)/1 -> Sum1/2
  Qf_0/1 -> Sum1/1
  Controller chosen/1 -> Sum/3
  Inertia compensation/1 -> Sum/1
  Core controller/3(Qcp) -> Controller chosen/4
  Core controller/2(Qcq) -> Controller chosen/3
  [controller] -> Supervisor/2(input)
  "T_d "/1 -> MATLAB Function/1(Td)
  [Rho] -> MATLAB Function/4(rho)
  [D] -> MATLAB Function/5(D)
  [eps_c] -> MATLAB Function/6(eps_c)
  [n_c] -> MATLAB Function/7(n_c)
  Constant1/1 -> Discrete Transfer Fcn/2
  Constant2/1 -> Discrete Transfer Fcn/3
  MATLAB Function/1(n_d) -> Discrete Transfer Fcn/1
  n/1 -> Supervisor/3(n), Core controller/3("n ")
  Discrete Transfer Fcn/1 -> Discrete Derivative/1, Core controller/1(n_r), Delay/1, Qff_0(nr)/1, Qff_1(nr)/1
  Acceleration limiter/1 -> Inertia compensation/1
  Supervisor/1(u) -> Memory/1
  Delay/1 -> MATLAB Function/8(n_r)
  [Kt4r] -> MATLAB Function/3(K_t0r)
  [Kt4f] -> MATLAB Function/2(K_t0)

== system ctrl_custom/Thruster control 1/Thruster 5/Propeller Hydrodynamics ==
  env : Inport
  n : Inport  Port=2
  Actual Force and Torque : MATLAB Function  TreatAsAtomicUnit=on
  Ta : Outport
  Qa : Outport  Port=2
  wires:
  n/1 -> Actual Force and Torque/1(n)
  [D] -> Actual Force and Torque/7(D)
  [Kq5f] -> Actual Force and Torque/2(Kq)
  Actual Force and Torque/2(Qa) -> Qa/1
  [Rho] -> Actual Force and Torque/6(Rho)
  env/1 -> Actual Force and Torque/9(env)
  [Kt5f] -> Actual Force and Torque/3(Kt)
  Actual Force and Torque/1(Ta) -> Ta/1
  [Kt5r] -> Actual Force and Torque/4(Ktr)
  [Kq5r] -> Actual Force and Torque/5(Kqr)
  [eps_c] -> Actual Force and Torque/8(eps_c)

== system ctrl_custom/Thruster control 1/Thruster 5/Shaft dynamics ==
  Qm : Inport
  Qa : Inport  Port=2
  Finding rotation speed : Gain  Gain=1/(2*pi*I_s)
  Integrator : Integrator  ExternalReset=either
  K_omega : Gain  Gain=K_omega*2*pi
  Sum : Sum  Inputs=-+-
  n : Outport
  wires:
  Qm/1 -> Sum/2
  Sum/1 -> Finding rotation speed/1
  Qa/1 -> Sum/1
  K_omega/1 -> Sum/3
  Finding rotation speed/1 -> Integrator/1
  Integrator/1 -> K_omega/1, n/1
  [reset] -> Integrator/2

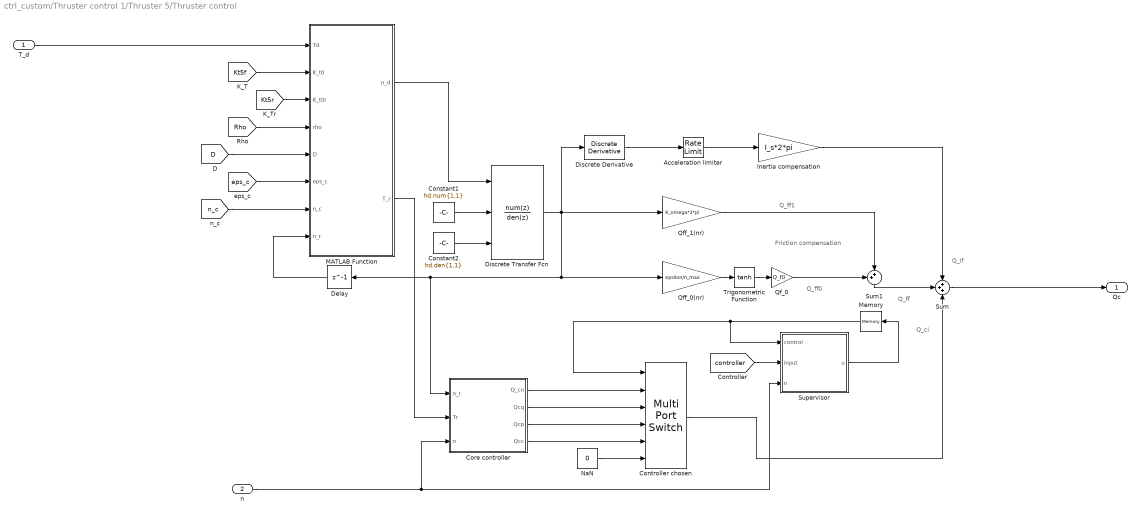
== system ctrl_custom/Thruster control 1/Thruster 5/Thruster control ==
  note: Q_ci
  note: Q_if
  note: Q_ff
  note: Q_ff0
  note: Q_ff1
  note: Friction compensation
  "T_d " : Inport
  n : Inport  Port=2
  Acceleration limiter : RateLimiter  RisingSlewLimit=Max_Acceleration  FallingSlewLimit=-Max_Acceleration  SampleTimeMode=inherited
  Constant1 : Constant  Value=hd.num{1,1}  VectorParams1D=off
  Constant2 : Constant  Value=hd.den{1,1}  VectorParams1D=off
  Controller chosen : MultiPortSwitch  Inputs=5
  Core controller : Subsystem
  Delay : Delay  DelayLength=1  InitialCondition=0
  Discrete Transfer Fcn : DiscreteTransferFcn  NumeratorSource=Input port  Numerator=[8.76e-05 0.0003481 8.648e-05]  DenominatorSource=Input port  Denominator=[1 -1.974 0.9746]  SampleTime=0.01  a0EqualsOne=on
      settings: InputPortMap=u0,p1,p3
  Discrete Derivative : simulink/Discrete/Discrete Derivative  gainval=1.0  ICPrevScaledInput=0.0  InputProcessing=Inherited  OutMin=[]  OutMax=[]  OutDataType=fixdt(1, 16)  OutScaling=2^-10  DoSatur=off
  Inertia compensation : Gain  Gain=I_s*2*pi
  MATLAB Function : MATLAB Function  TreatAsAtomicUnit=on
  Memory : Memory  X0=1
  NaN : Constant  Value=0
  Qf_0 : Gain  Gain=Q_f0
  Qff_0(nr) : Gain  Gain=epsilon/n_max
  Qff_1(nr) : Gain  Gain=K_omega*2*pi
  Sum : Sum  Inputs=+++
  Sum1 : Sum  Inputs=++|
  Supervisor : MATLAB Function  TreatAsAtomicUnit=on
  Trigonometric Function : Trigonometry  Operator=tanh
  Qc : Outport
  wires:
  Sum/1 -> Qc/1
  MATLAB Function/2(T_r) -> Core controller/2("Tr ")
  Discrete Derivative/1 -> Acceleration limiter/1
  Qff_0(nr)/1 -> Trigonometric Function/1
  Trigonometric Function/1 -> Qf_0/1
  Sum1/1 -> Sum/2
  Core controller/1(Q_cn) -> Controller chosen/2
  Core controller/4(Qcc) -> Controller chosen/5
  NaN/1 -> Controller chosen/6
  Memory/1 -> Supervisor/1(control), Controller chosen/1
  Qff_1(nr)/1 -> Sum1/2
  Qf_0/1 -> Sum1/1
  Controller chosen/1 -> Sum/3
  Inertia compensation/1 -> Sum/1
  Core controller/3(Qcp) -> Controller chosen/4
  Core controller/2(Qcq) -> Controller chosen/3
  [controller] -> Supervisor/2(input)
  "T_d "/1 -> MATLAB Function/1(Td)
  [Rho] -> MATLAB Function/4(rho)
  [D] -> MATLAB Function/5(D)
  [eps_c] -> MATLAB Function/6(eps_c)
  [n_c] -> MATLAB Function/7(n_c)
  Constant1/1 -> Discrete Transfer Fcn/2
  Constant2/1 -> Discrete Transfer Fcn/3
  MATLAB Function/1(n_d) -> Discrete Transfer Fcn/1
  Discrete Transfer Fcn/1 -> Discrete Derivative/1, Qff_0(nr)/1, Core controller/1(n_r), Delay/1, Qff_1(nr)/1
  Acceleration limiter/1 -> Inertia compensation/1
  Supervisor/1(u) -> Memory/1
  Delay/1 -> MATLAB Function/8(n_r)
  n/1 -> Core controller/3("n "), Supervisor/3(n)
  [Kt5r] -> MATLAB Function/3(K_t0r)
  [Kt5f] -> MATLAB Function/2(K_t0)

== system ctrl_custom/Thruster control 1/Thruster 6/Propeller Hydrodynamics ==
  env : Inport
  n : Inport  Port=2
  Actual Force and Torque : MATLAB Function  TreatAsAtomicUnit=on
  Ta : Outport
  Qa : Outport  Port=2
  wires:
  n/1 -> Actual Force and Torque/1(n)
  [D] -> Actual Force and Torque/7(D)
  [Kq6f] -> Actual Force and Torque/2(Kq)
  Actual Force and Torque/2(Qa) -> Qa/1
  [Rho] -> Actual Force and Torque/6(Rho)
  env/1 -> Actual Force and Torque/9(env)
  [Kt6f] -> Actual Force and Torque/3(Kt)
  Actual Force and Torque/1(Ta) -> Ta/1
  [Kt6r] -> Actual Force and Torque/4(Ktr)
  [Kq6r] -> Actual Force and Torque/5(Kqr)
  [eps_c] -> Actual Force and Torque/8(eps_c)

== system ctrl_custom/Thruster control 1/Thruster 6/Shaft dynamics ==
  Qm : Inport
  Qa : Inport  Port=2
  Finding rotation speed : Gain  Gain=1/(2*pi*I_s)
  Integrator : Integrator  ExternalReset=either
  K_omega : Gain  Gain=K_omega*2*pi
  Sum : Sum  Inputs=-+-
  n : Outport
  wires:
  Qm/1 -> Sum/2
  Sum/1 -> Finding rotation speed/1
  Qa/1 -> Sum/1
  K_omega/1 -> Sum/3
  Integrator/1 -> K_omega/1, n/1
  [reset] -> Integrator/2
  Finding rotation speed/1 -> Integrator/1

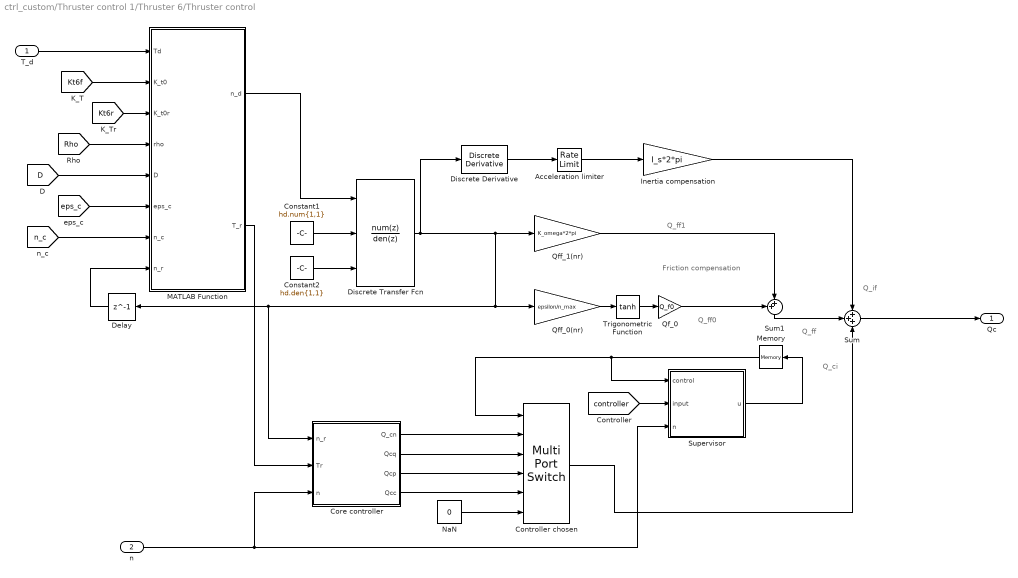
== system ctrl_custom/Thruster control 1/Thruster 6/Thruster control ==
  note: Q_ci
  note: Q_if
  note: Q_ff
  note: Q_ff0
  note: Q_ff1
  note: Friction compensation
  "T_d " : Inport
  n : Inport  Port=2
  Acceleration limiter : RateLimiter  RisingSlewLimit=Max_Acceleration  FallingSlewLimit=-Max_Acceleration  SampleTimeMode=inherited
  Constant1 : Constant  Value=hd.num{1,1}  VectorParams1D=off
  Constant2 : Constant  Value=hd.den{1,1}  VectorParams1D=off
  Controller chosen : MultiPortSwitch  Inputs=5
  Core controller : Subsystem
  Delay : Delay  DelayLength=1  InitialCondition=0
  Discrete Transfer Fcn : DiscreteTransferFcn  NumeratorSource=Input port  Numerator=[8.76e-05 0.0003481 8.648e-05]  DenominatorSource=Input port  Denominator=[1 -1.974 0.9746]  SampleTime=0.01  a0EqualsOne=on
      settings: InputPortMap=u0,p1,p3
  Discrete Derivative : simulink/Discrete/Discrete Derivative  gainval=1.0  ICPrevScaledInput=0.0  InputProcessing=Inherited  OutMin=[]  OutMax=[]  OutDataType=fixdt(1, 16)  OutScaling=2^-10  DoSatur=off
  Inertia compensation : Gain  Gain=I_s*2*pi
  MATLAB Function : MATLAB Function  TreatAsAtomicUnit=on
  Memory : Memory  X0=1
  NaN : Constant  Value=0
  Qf_0 : Gain  Gain=Q_f0
  Qff_0(nr) : Gain  Gain=epsilon/n_max
  Qff_1(nr) : Gain  Gain=K_omega*2*pi
  Sum : Sum  Inputs=+++
  Sum1 : Sum  Inputs=++|
  Supervisor : MATLAB Function  TreatAsAtomicUnit=on
  Trigonometric Function : Trigonometry  Operator=tanh
  Qc : Outport
  wires:
  Sum/1 -> Qc/1
  MATLAB Function/2(T_r) -> Core controller/2("Tr ")
  Discrete Derivative/1 -> Acceleration limiter/1
  Qff_0(nr)/1 -> Trigonometric Function/1
  Trigonometric Function/1 -> Qf_0/1
  Sum1/1 -> Sum/2
  Core controller/1(Q_cn) -> Controller chosen/2
  Core controller/4(Qcc) -> Controller chosen/5
  NaN/1 -> Controller chosen/6
  Memory/1 -> Supervisor/1(control), Controller chosen/1
  Qff_1(nr)/1 -> Sum1/2
  Qf_0/1 -> Sum1/1
  Controller chosen/1 -> Sum/3
  Inertia compensation/1 -> Sum/1
  Core controller/3(Qcp) -> Controller chosen/4
  Core controller/2(Qcq) -> Controller chosen/3
  [controller] -> Supervisor/2(input)
  "T_d "/1 -> MATLAB Function/1(Td)
  [Rho] -> MATLAB Function/4(rho)
  [D] -> MATLAB Function/5(D)
  [eps_c] -> MATLAB Function/6(eps_c)
  [n_c] -> MATLAB Function/7(n_c)
  Constant1/1 -> Discrete Transfer Fcn/2
  Constant2/1 -> Discrete Transfer Fcn/3
  MATLAB Function/1(n_d) -> Discrete Transfer Fcn/1
  n/1 -> Supervisor/3(n), Core controller/3("n ")
  Discrete Transfer Fcn/1 -> Discrete Derivative/1, Core controller/1(n_r), Delay/1, Qff_0(nr)/1, Qff_1(nr)/1
  Acceleration limiter/1 -> Inertia compensation/1
  Supervisor/1(u) -> Memory/1
  Delay/1 -> MATLAB Function/8(n_r)
  [Kt6r] -> MATLAB Function/3(K_t0r)
  [Kt6f] -> MATLAB Function/2(K_t0)

== system ctrl_custom/Thruster control 1/Thruster 1/Thruster control/Core controller ==
  note: Core controller: Shaft speed
  n_r : Inport
  "Tr " : Inport  Port=2
  "n " : Inport  Port=3
  Core controller: Torque,Power and Combined Torque/Power : MATLAB Function  TreatAsAtomicUnit=on
  Integrator : Integrator  ExternalReset=either  UpperSaturationLimit=Q_max  LowerSaturationLimit=-Q_max
  Ki : Gain  Gain=Kp/0.05
  Kp : Gain  Gain=Kp
  Sum : Sum  Inputs=+|-
  Sum1 : Sum  Inputs=|++
  reset : S-Function  Priority=1  FunctionName=NIVeriStandIO  Parameters=width dtype portnum stime stype btype  SFunctionDeploymentMode=off  EnableBusSupport=off  mask(NI VeriStand Inport){portnum=1, width=-1, stime=-1, dtype=auto, stype=auto, btype=1}
      mask prompts: portnum "Port number:"; width "Port dimensions (-1 for dynamically sized):"; stime "Sample time (-1 for inherited):"; dtype "Data type:"; stype "Signal type:"; btype "Block type:"
      mask help: Use this inport on any level of nested subsystems to allow NI VeriStand software to map signals to it.
      mask init:
      | NIVeriStandIO_init;
      settings: CopyFcn=NIVeriStand_MDL_functions('', 'IO_copy');  DeleteFcn=NIVeriStand_MDL_functions('', 'IO_delete');  MoveFcn=set_param(gcb, 'Mask', 'on');
      mask Callback portnum: NIVeriStand_MDL_functions('', 'IO_setportnum');
      mask TypeOptions dtype: auto | double | single | int8 | uint8 | int16 | uint16 | int32 | uint32 | boolean
      mask Callback dtype: NIVeriStand_MDL_functions('', 'IO_booleansignal');
      mask TypeOptions stype: auto | real | complex
      mask Display:
      | patch([-x x], [-y y], [.90980 .81960 .32156]);
      | plot([xrad -x x xrad], [yrad -y y yrad]);
      | fprintf('NI In%d', portnum);
  Q_cn : Outport
  Qcq : Outport  Port=2
  Qcp : Outport  Port=3
  Qcc : Outport  Port=4
  wires:
  [k_cc] -> Core controller: Torque,Power and Combined Torque/Power/1(k_cc)
  [p_cc] -> Core controller: Torque,Power and Combined Torque/Power/2(p_cc)
  [r_cc] -> Core controller: Torque,Power and Combined Torque/Power/3(r_cc)
  Core controller: Torque,Power and Combined Torque/Power/3(Qcc) -> Qcc/1
  [Kt1f] -> Core controller: Torque,Power and Combined Torque/Power/5(K_t0)
  [D] -> Core controller: Torque,Power and Combined Torque/Power/7(D)
  [Kq1f] -> Core controller: Torque,Power and Combined Torque/Power/6(K_q0)
  [Rho] -> Core controller: Torque,Power and Combined Torque/Power/9(rho)
  "n "/1 -> Sum/2, Core controller: Torque,Power and Combined Torque/Power/4(n)
  "Tr "/1 -> Core controller: Torque,Power and Combined Torque/Power/8(Tr)
  Core controller: Torque,Power and Combined Torque/Power/2(Qcp) -> Qcp/1
  Core controller: Torque,Power and Combined Torque/Power/1(Qcq) -> Qcq/1
  n_r/1 -> Sum/1
  Ki/1 -> Integrator/1
  Kp/1 -> Sum1/1
  Integrator/1 -> Sum1/2
  Sum1/1 -> Q_cn/1
  Sum/1 -> Ki/1, Kp/1
  reset/1 -> Integrator/2
  [eps_c] -> Core controller: Torque,Power and Combined Torque/Power/10(eps_c)
  [Kt1r] -> Core controller: Torque,Power and Combined Torque/Power/11(K_t0r)
  [Kq1r] -> Core controller: Torque,Power and Combined Torque/Power/12(K_q0r)
